simulink model "variableStiffnessJoint"  (R2018a)
settings: Solver=VariableStepAuto  StartTime=0.0  StopTime=10.0  RelTol=1e-3
settings Model: Creator=pei-T  LastModifiedBy=pei-T

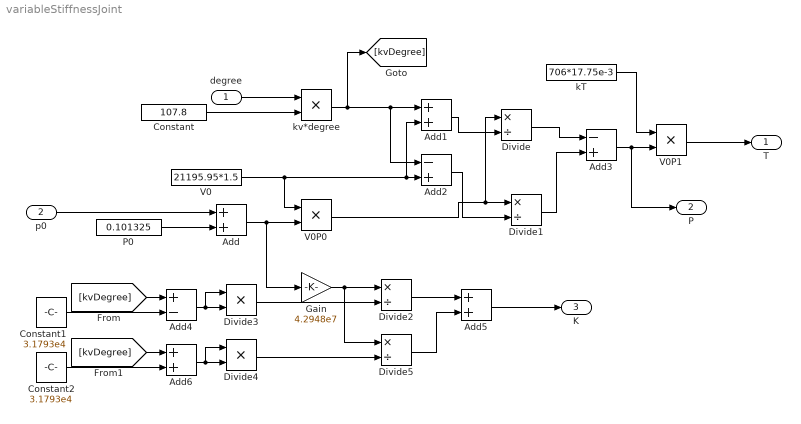
== system variableStiffnessJoint ==
  degree : Inport
  p0 : Inport  Port=2
  Add{,1,5..6} (4 alike) : Sum
  Add2 : Sum  Inputs=-+
  Add3 : Sum  Inputs=-+
  Add4 : Sum  Inputs=+-
  Constant : Constant  Value=107.8
  Constant1 : Constant  Value=3.1793e4
  Constant2 : Constant  Value=3.1793e4
  Divide{,1..2,5} (4 alike) : Product  Inputs=*/
  Divide3 : Product  Inputs=**
  Divide4 : Product  Inputs=**
  Gain : Gain  Gain=4.2948e7
  P0 : Constant  Value=0.101325
  V0 : Constant  Value=21195.95*1.5
  V0P0 : Product
  V0P1 : Product
  kT : Constant  Value=706*17.75e-3
  kv*degree : Product
  T : Outport
  P : Outport  Port=2
  K : Outport  Port=3
  wires:
  Divide4/1 -> Divide5/2
  Divide5/1 -> Add5/2
  Divide3/1 -> Divide2/2
  [kvDegree] -> Add6/1
  Add5/1 -> K/1
  Divide/1 -> Add3/1
  kT/1 -> V0P1/1
  kv*degree/1 -> [kvDegree], Add2/1, Add1/1
  degree/1 -> kv*degree/1
  P0/1 -> Add/2
  Constant/1 -> kv*degree/2
  V0P1/1 -> T/1
  V0/1 -> V0P0/1, Add2/2, Add1/2
  [kvDegree] -> Add4/1
  Divide2/1 -> Add5/1
  Add6/1 -> Divide4/1, Divide4/2
  Constant2/1 -> Add6/2
  Divide1/1 -> Add3/2
  Add/1 -> Gain/1, V0P0/2
  Constant1/1 -> Add4/2
  Add3/1 -> P/1, V0P1/2
  Gain/1 -> Divide5/1, Divide2/1
  p0/1 -> Add/1
  Add1/1 -> Divide/2
  Add4/1 -> Divide3/1, Divide3/2
  V0P0/1 -> Divide1/1, Divide/1
  Add2/1 -> Divide1/2
